simulink model "drone_main_dynamixal"  (R2023b)
settings: Solver=FixedStepAuto  StartTime=0.0  StopTime=inf  FixedStep=0.001  RelTol=1e-3
model workspace: external: MATLAB File drone_DataFile.m (data not in the file)
values from neighbouring files (symbols this model uses):
  coefthrust = 5.7199 / (max_prop^2)    (= 5.7199e-06)    [parameters.m]    (also in parameters.mat)
  coeftorque = 0.4008 / (max_prop^2)    (= 4.008e-07)    [parameters.m]    (also in parameters.mat)
  controlmatrix = pinv(controlmatrix)    [parameters.m]    (also in parameters.mat = [121408.493932 121408.493932 -121408.493932 -121408.493932 -)
  g = 9.8067    [parameters.m]    (also in parameters.mat)
  I = [0.0283    0.0003    0.0072 ... (first row only)    [parameters.m]    (also in parameters.mat = [0.0283  0.0003  0.0072; 0.0003  0.521  -0.0001; 0.0072  -0.)
  M =     [parameters.mat]
  m = pinv(mixmatrix)*b    [test.m]
  max_prop = 1000    [parameters.m]    (also in parameters.mat)
  poly_traj = pTraj    [trajectory.m]
  route = [0 0 1 0.5*pi ... (first row only)    [parameters.m]    (also in parameters.mat = [0 0 -3 -3 -3 3 0 3 3 4 4 4 ... (24 elements, 6x4)])
  smiData = struct    [drone_DataFile.m]
  total_mass = 2.1309    [parameters.m]    (also in parameters.mat)
undefined symbols (not defined in the file or in its folder): mass_total, X, Y, Z
libraries: sm_lib x173, slpidlib x90, nesl_utility x72, fl_lib x32, slctrl_autotuning x21, quadcopter_library x8, sdl_lib x8, simulink x3
(part 1 of 19)
settings Model: Creator=karl  LastModifiedBy=karl
settings SolverCC: ZeroCrossAlgorithm=Adaptive
settings DebuggingCC: MaskedZcDiagnostic=none  IgnoredZcDiagnostic=none
settings ExplorerConfigSet: InternalSimMechanicsExplorerSettings="<ExplorerConfiguration><canonicalview>default</canonicalview><AnimationSetting><BasePlaybackSpeed>1.0</BasePlaybackSpeed><PlaybackSpeedFactor>1.0</PlaybackSpeedFactor></AnimationSetting><TilePanel><TileInfo><Tiles Columns=\"1\" Count=\"1\" Rows=\"1\"><Column Weight=\"1\"/><Row Weight=\"1\"/><Tile Height=\"1\" Width=\"1\" X=\"0\" Y=\"0\"/></Tiles></TileInfo><SceneInfo><SceneViewer><BGColor><R>0.60000002384185791</R><G>0.60000002384185791</G><B>0.60000002384185791</B></BGColor><Camera><DoPerspective>on</DoPerspective><Position><X>2.81198467739789759</X><Y>2.16442511828485351</Y><Z>2.00493354781460198</Z></Position><Center><X>3.04927914831391655</X><Y>4.00827432510628157</Y><Z>0.998712364972069055</Z></Center><Up><X>0</X><Y>-2.22044604925031308e-16</Y><Z>1</Z></Up><ViewLimDist>1</ViewLimDist><YLim>0.466307658154998583</YLim><XLim>0.670479471373142677</XLim></Camera></SceneViewer></SceneInfo></TilePanel><MechEditorPanel><Cameras><Camera><Id>Camera1</Id><Value><Name>Camera1</Name><NativeCamera><PositionTrackingFeature>plant.camera_Frame.R</PositionTrackingFeature><CenterTrackingFeature>plant.centerbody.F6</CenterTrackingFeature><UpVectorTrackingFeature>plant.Cartesian_Joint.F</UpVectorTrackingFeature><CenterTrackingOrigin>on</CenterTrackingOrigin><UpVectorTrackingDirection>-Y</UpVectorTrackingDirection></NativeCamera></Value></Camera></Cameras><GfxPanelCameraMap><MapElement CameraMLId=\"Camera1\" GfxPanelIndex=\"0\"/></GfxPanelCameraMap><VideoCreator><PlaybackSpeedRatio>1.0</PlaybackSpeedRatio><FrameRate>60</FrameRate><VideoFormat>MPEG-4</VideoFormat><FrameSize>[1920 1080]</FrameSize></VideoCreator></MechEditorPanel></ExplorerConfiguration>"

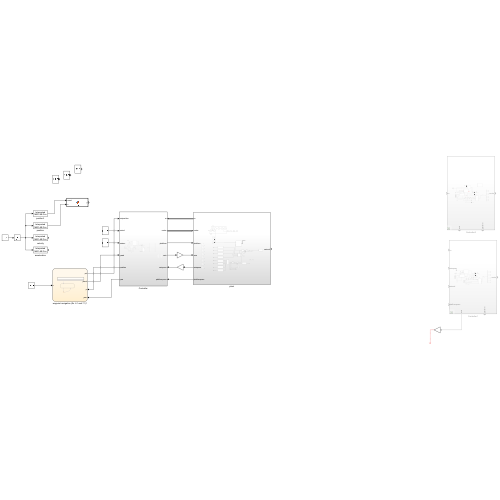
[thumbnail: Simulink's stored preview of the top-level diagram]
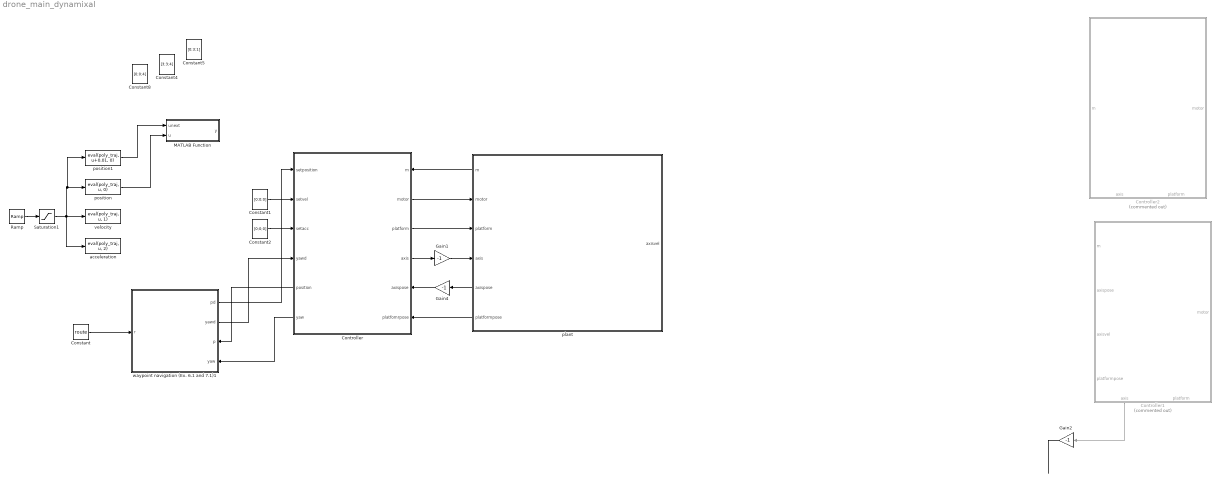
== system drone_main_dynamixal ==
  Constant : Constant  Value=route
  Constant1 : Constant  Value=[0;0;0]
  Constant2 : Constant  Value=[0;0;0]
  Constant4 : Constant  Value=[3;3;4]
  Constant5 : Constant  Value=[0;3;1]
  Constant8 : Constant  Value=[0;0;4]
  Controller : Subsystem
      settings: PortSchema="{\"entries\":[{\"content\":{\"sides\":[{\"content\":{\"connectorIds\":[\"In1\",\"In2\",\"In3\",\"In4\",\"Out4\",\"Out5\"]},\"type\":\"ConnectorPlacement.EquallySpacedRectSide\",\"uuid\":\"efd116df-0710-4bc4-bd30-46d2282b54a0\"},{\"content\":{\"connectorIds\":[\"In5\",\"Out1\",\"Out2\",\"Out3\",\"In6\",\"In7\"],\"side\":\"RIGHT\"},\"type\":\"ConnectorPlacement.EquallySpacedRectSide\",\"uuid\":\"42a0262b-89db-4dee-9ad3-14016f8ac5f1\"},{\"content\":{\"side\":\"TOP\"},\"type\":\"ConnectorPlacement.EquallySpacedRectSide\",\"uuid\":\"e37570b1-13d5-473e-a4a2-7c37e0d0ffe3\"},{\"content\":{\"side\":\"BOTTOM\"},\"type\":\"ConnectorPlacement.EquallySpacedRectSide\",\"uuid\":\"fd86b602-742f-417b-a2c4-bd46caad86d3\"}]},\"type\":\"ConnectorPlacement.EquallySpacedConnector\",\"uuid\":\"c2e19d15-eb80-41e4-99c2-17f1e388988e\"}],\"packageUris\":[\"http://schema.mathworks.com/mf0/Connector/R2020b\"],\"version\":\"1.0\"}"
  Controller1 : Subsystem  Commented=on
      settings: PortSchema="{\"entries\":[{\"content\":{\"sides\":[{\"content\":{\"connectorIds\":[\"In1\",\"In2\",\"In3\",\"In4\"]},\"type\":\"ConnectorPlacement.EquallySpacedRectSide\",\"uuid\":\"efd116df-0710-4bc4-bd30-46d2282b54a0\"},{\"content\":{\"connectorIds\":[\"Out1\"],\"side\":\"RIGHT\"},\"type\":\"ConnectorPlacement.EquallySpacedRectSide\",\"uuid\":\"42a0262b-89db-4dee-9ad3-14016f8ac5f1\"},{\"content\":{\"side\":\"TOP\"},\"type\":\"ConnectorPlacement.EquallySpacedRectSide\",\"uuid\":\"e37570b1-13d5-473e-a4a2-7c37e0d0ffe3\"},{\"content\":{\"connectorIds\":[\"Out2\",\"Out3\"],\"side\":\"BOTTOM\"},\"type\":\"ConnectorPlacement.EquallySpacedRectSide\",\"uuid\":\"fd86b602-742f-417b-a2c4-bd46caad86d3\"}]},\"type\":\"ConnectorPlacement.EquallySpacedConnector\",\"uuid\":\"c2e19d15-eb80-41e4-99c2-17f1e388988e\"}],\"packageUris\":[\"http://schema.mathworks.com/mf0/Connector/R2020b\"],\"version\":\"1.0\"}"
  Controller2 : Subsystem  Commented=on
      settings: PortSchema="{\"entries\":[{\"content\":{\"sides\":[{\"content\":{\"connectorIds\":[\"In1\"]},\"type\":\"ConnectorPlacement.EquallySpacedRectSide\",\"uuid\":\"efd116df-0710-4bc4-bd30-46d2282b54a0\"},{\"content\":{\"connectorIds\":[\"Out1\"],\"side\":\"RIGHT\"},\"type\":\"ConnectorPlacement.EquallySpacedRectSide\",\"uuid\":\"42a0262b-89db-4dee-9ad3-14016f8ac5f1\"},{\"content\":{\"side\":\"TOP\"},\"type\":\"ConnectorPlacement.EquallySpacedRectSide\",\"uuid\":\"e37570b1-13d5-473e-a4a2-7c37e0d0ffe3\"},{\"content\":{\"connectorIds\":[\"Out2\",\"Out3\"],\"side\":\"BOTTOM\"},\"type\":\"ConnectorPlacement.EquallySpacedRectSide\",\"uuid\":\"fd86b602-742f-417b-a2c4-bd46caad86d3\"}]},\"type\":\"ConnectorPlacement.EquallySpacedConnector\",\"uuid\":\"c2e19d15-eb80-41e4-99c2-17f1e388988e\"}],\"packageUris\":[\"http://schema.mathworks.com/mf0/Connector/R2020b\"],\"version\":\"1.0\"}"
  Gain1 : Gain  Gain=-1
  Gain2 : Gain  Gain=-1
  Gain4 : Gain  Gain=-1
  MATLAB Function : MATLAB Function  TreatAsAtomicUnit=on
  Ramp : simulink/Sources/Ramp  slope=1  start=0  InitialOutput=0
  Saturation1 : Saturate  UpperLimit=knots(end)  LowerLimit=0
  acceleration : MATLABFcn  MATLABFcn=eval(poly_traj, u, 2)  OutputDimensions=[3 1]  Output1D=off
  plant : Subsystem
      settings: PortSchema="{\"entries\":[{\"content\":{\"sides\":[{\"content\":{\"connectorIds\":[\"Out2\",\"In1\",\"In2\",\"In3\",\"Out3\",\"Out4\"]},\"type\":\"ConnectorPlacement.EquallySpacedRectSide\",\"uuid\":\"1c064c66-4770-46ed-8bde-fcd9daa0cfea\"},{\"content\":{\"connectorIds\":[\"Out1\"],\"side\":\"RIGHT\"},\"type\":\"ConnectorPlacement.EquallySpacedRectSide\",\"uuid\":\"2bc9ec3c-f7fe-448b-b9a0-aabfb7a731b3\"},{\"content\":{\"side\":\"TOP\"},\"type\":\"ConnectorPlacement.EquallySpacedRectSide\",\"uuid\":\"776f5a84-0136-4a0a-add1-2781f8ebe025\"},{\"content\":{\"side\":\"BOTTOM\"},\"type\":\"ConnectorPlacement.EquallySpacedRectSide\",\"uuid\":\"8fe710a9-ef9a-4b6e-99e6-9612389d5d8d\"}]},\"type\":\"ConnectorPlacement.EquallySpacedConnector\",\"uuid\":\"c1b0af6b-0af1-4f81-9887-9b2d00ee34a0\"}],\"packageUris\":[\"http://schema.mathworks.com/mf0/Connector/R2020b\"],\"version\":\"1.0\"}"
  position : MATLABFcn  MATLABFcn=eval(poly_traj, u, 0)  OutputDimensions=[3 1]  Output1D=off
  position1 : MATLABFcn  MATLABFcn=eval(poly_traj, u+0.01, 0)  OutputDimensions=[3 1]  Output1D=off
  velocity : MATLABFcn  MATLABFcn=eval(poly_traj, u, 1)  OutputDimensions=[3 1]  Output1D=off
  waypoint navigation (Ex. 6.1 and 7.1)1 : Stateflow chart  TreatAsAtomicUnit=on
      settings: PortSchema="{\"entries\":[{\"content\":{\"sides\":[{\"content\":{\"connectorIds\":[\"In1\"]},\"type\":\"ConnectorPlacement.EquallySpacedRectSide\",\"uuid\":\"7c2fff0d-1179-4786-9432-1971d7acd904\"},{\"content\":{\"connectorIds\":[\"Out2\",\"Out1\",\"In3\",\"In2\"],\"side\":\"RIGHT\"},\"type\":\"ConnectorPlacement.EquallySpacedRectSide\",\"uuid\":\"377a8206-b310-41c0-9a17-faf5318c89cb\"},{\"content\":{\"side\":\"TOP\"},\"type\":\"ConnectorPlacement.EquallySpacedRectSide\",\"uuid\":\"b953090a-ffdb-4e30-a5fe-7bef9655f1cf\"},{\"content\":{\"side\":\"BOTTOM\"},\"type\":\"ConnectorPlacement.EquallySpacedRectSide\",\"uuid\":\"03dc7a24-529e-4020-b953-d1c4751c5c80\"}]},\"type\":\"ConnectorPlacement.EquallySpacedConnector\",\"uuid\":\"03bac9f4-6480-492d-9af3-57aec4db8fd8\"}],\"packageUris\":[\"http://schema.mathworks.com/mf0/Connector/R2020b\"],\"version\":\"1.0\"}"
  wires:
  plant/2(m) -> Controller/5(m)
  Controller/2(platform) -> plant/2(platform)
  Controller/3(axis) -> Gain1/1
  Gain1/1 -> plant/3(axis)
  Controller/1(motor) -> plant/1(motor)
  Controller1/2(axis) -> Gain2/1
  Gain2/1 -> ?
  plant/3(axispose) -> Gain4/1
  Gain4/1 -> Controller/6(axispose)
  plant/4(platformpose) -> Controller/7(platfomrpose)
  Constant/1 -> waypoint navigation (Ex. 6.1 and 7.1)1/1(r)
  position/1 -> MATLAB Function/2(u)
  Controller/4(position) -> waypoint navigation (Ex. 6.1 and 7.1)1/3(p)
  waypoint navigation (Ex. 6.1 and 7.1)1/1(yawd) -> Controller/4(yawd)
  Controller/5(yaw) -> waypoint navigation (Ex. 6.1 and 7.1)1/2(yaw)
  Saturation1/1 -> acceleration/1, position1/1, position/1, velocity/1
  Ramp/1 -> Saturation1/1
  position1/1 -> MATLAB Function/1(unext)
  Constant1/1 -> Controller/2(setvel)
  Constant2/1 -> Controller/3(setacc)
  waypoint navigation (Ex. 6.1 and 7.1)1/2(pd) -> Controller/1(setposition)

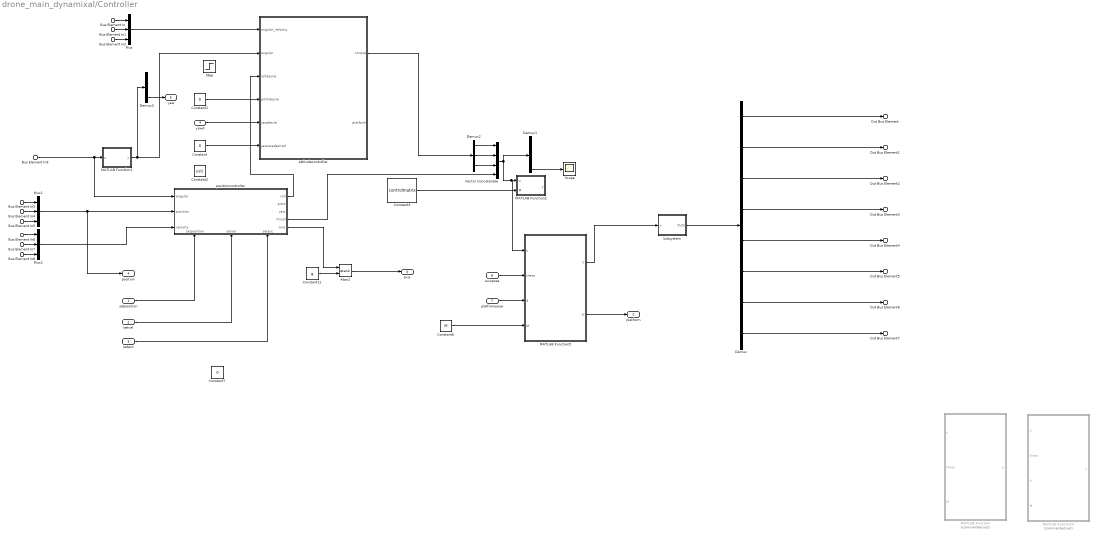
== system drone_main_dynamixal/Controller ==
  setposition : Inport
  setvel : Inport  Port=2
  setacc : Inport  Port=3
  yawd : Inport  Port=4
  Bus Element In : Inport  Port=5  PortName=m  Element=nRoll
  Bus Element In1 : Inport  Port=5  PortName=m  Element=nPitch
  Bus Element In2 : Inport  Port=5  PortName=m  Element=nYaw
  Bus Element In3 : Inport  Port=5  PortName=m  Element=px
  Bus Element In4 : Inport  Port=5  PortName=m  Element=py
  Bus Element In5 : Inport  Port=5  PortName=m  Element=pz
  Bus Element In6 : Inport  Port=5  PortName=m  Element=vx
  Bus Element In7 : Inport  Port=5  PortName=m  Element=vy
  Bus Element In8 : Inport  Port=5  PortName=m  Element=vz
  Bus Element In9 : Inport  Port=5  PortName=m  Element=R
  axispose : Inport  Port=6
  platfomrpose : Inport  Port=7
  Atan2 : Trigonometry  Operator=atan2
  Constant : Constant  Value=0
  Constant1 : Constant  Value=0
  Constant11 : Constant  Value=g
  Constant2 : Constant  Value=pi/2
  Constant3 : Constant  Value=controlmatrix
  Constant6 : Constant  Value=M  OutDataTypeStr=Bus: M_bus
  Constant7 : Constant  Value=0
  Demux : Demux  Outputs=8
  Demux1 : Demux
  Demux2 : Demux  Outputs=3
  Demux3 : Demux  Outputs=3
  MATLAB Function : MATLAB Function  Commented=on  TreatAsAtomicUnit=on
  MATLAB Function1 : MATLAB Function  TreatAsAtomicUnit=on
  MATLAB Function2 : MATLAB Function  TreatAsAtomicUnit=on
  MATLAB Function4 : MATLAB Function  Commented=on  TreatAsAtomicUnit=on
  MATLAB Function5 : MATLAB Function  TreatAsAtomicUnit=on
  Mux : Mux  Inputs=3
  Mux1 : Mux  Inputs=3
  Mux2 : Mux  Inputs=3
  Scope : Scope
  Step : Step  SampleTime=0
  Subsystem : Subsystem
  Vector Concatenate : Concatenate  NumInputs=4
  attitudecontroller : Subsystem
  positioncontroller : Subsystem
      settings: PortSchema="{\"entries\":[{\"content\":{\"sides\":[{\"content\":{\"connectorIds\":[\"In1\",\"In2\",\"In3\"]},\"type\":\"ConnectorPlacement.EquallySpacedRectSide\",\"uuid\":\"8fc0619c-da24-474a-ba81-4a0e6403e529\"},{\"content\":{\"connectorIds\":[\"Out1\",\"Out2\",\"Out3\",\"Out4\",\"Out5\"],\"side\":\"RIGHT\"},\"type\":\"ConnectorPlacement.EquallySpacedRectSide\",\"uuid\":\"3b7bf8fd-1c12-492b-bf3d-80eeb1c43df6\"},{\"content\":{\"side\":\"TOP\"},\"type\":\"ConnectorPlacement.EquallySpacedRectSide\",\"uuid\":\"d4c65c09-2611-4b76-817c-4c3799ca9b05\"},{\"content\":{\"connectorIds\":[\"In4\",\"In5\",\"In6\"],\"side\":\"BOTTOM\"},\"type\":\"ConnectorPlacement.EquallySpacedRectSide\",\"uuid\":\"94af8736-882f-4d33-beaa-402d25cea3b1\"}]},\"type\":\"ConnectorPlacement.EquallySpacedConnector\",\"uuid\":\"0c77d207-25a9-4738-a568-946a6093f630\"}],\"packageUris\":[\"http://schema.mathworks.com/mf0/Connector/R2020b\"],\"version\":\"1.0\"}"
  Out Bus Element : Outport  PortName=motor  Element=Output
  Out Bus Element1 : Outport  PortName=motor  Element=Output1
  Out Bus Element2 : Outport  PortName=motor  Element=Output2
  Out Bus Element3 : Outport  PortName=motor  Element=Output3
  Out Bus Element4 : Outport  PortName=motor  Element=Output4
  Out Bus Element5 : Outport  PortName=motor  Element=Output5
  Out Bus Element6 : Outport  PortName=motor  Element=Output6
  Out Bus Element7 : Outport  PortName=motor  Element=Output7
  platform : Outport  Port=2
  axis : Outport  Port=3
  position : Outport  Port=4
  yaw : Outport  Port=5
  wires:
  Constant3/1 -> MATLAB Function2/2(M)
  Vector Concatenate/1 -> MATLAB Function5/1(u), MATLAB Function2/1(u), Demux1/1
  Bus Element In9/1 -> positioncontroller/1(angular), MATLAB Function1/1(u)
  Subsystem/1(Out1) -> Demux/1
  Mux1/1 -> position/1, positioncontroller/2(position)
  setposition/1 -> positioncontroller/4(setposition)
  Mux/1 -> attitudecontroller/1(angular_velocity)
  attitudecontroller/1(torque) -> Demux2/1
  yawd/1 -> attitudecontroller/5(yawdesire)
  Demux1/4 -> Scope/1
  positioncontroller/4(thrust) -> Vector Concatenate/4
  positioncontroller/1(roll) -> attitudecontroller/3(rolldesire)
  Constant1/1 -> attitudecontroller/4(pitchdesire)
  Mux2/1 -> positioncontroller/3(velocity)
  Bus Element In/1 -> Mux/1
  Bus Element In1/1 -> Mux/2
  Bus Element In2/1 -> Mux/3
  Bus Element In4/1 -> Mux1/2
  Bus Element In5/1 -> Mux1/3
  Bus Element In3/1 -> Mux1/1
  Bus Element In6/1 -> Mux2/1
  Bus Element In8/1 -> Mux2/3
  Bus Element In7/1 -> Mux2/2
  MATLAB Function1/1(y) -> Demux3/1, attitudecontroller/2(angular)
  Demux2/2 -> Vector Concatenate/2
  Demux2/1 -> Vector Concatenate/1
  Demux2/3 -> Vector Concatenate/3
  MATLAB Function5/1(y) -> Subsystem/1(y)
  Constant11/1 -> Atan2/2
  Constant6/1 -> MATLAB Function5/4(M)
  positioncontroller/5(axis) -> Atan2/1
  Constant/1 -> attitudecontroller/6(yawratedesired)
  MATLAB Function5/2(p) -> platform/1
  platfomrpose/1 -> MATLAB Function5/3(d)
  axispose/1 -> MATLAB Function5/2(theta)
  Demux3/3 -> yaw/1
  setacc/1 -> positioncontroller/6(setacc)
  setvel/1 -> positioncontroller/5(setvel)
  Atan2/1 -> axis/1
  Demux/1 -> Out Bus Element/1
  Demux/2 -> Out Bus Element1/1
  Demux/4 -> Out Bus Element3/1
  Demux/3 -> Out Bus Element2/1
  Demux/5 -> Out Bus Element4/1
  Demux/6 -> Out Bus Element5/1
  Demux/7 -> Out Bus Element6/1
  Demux/8 -> Out Bus Element7/1

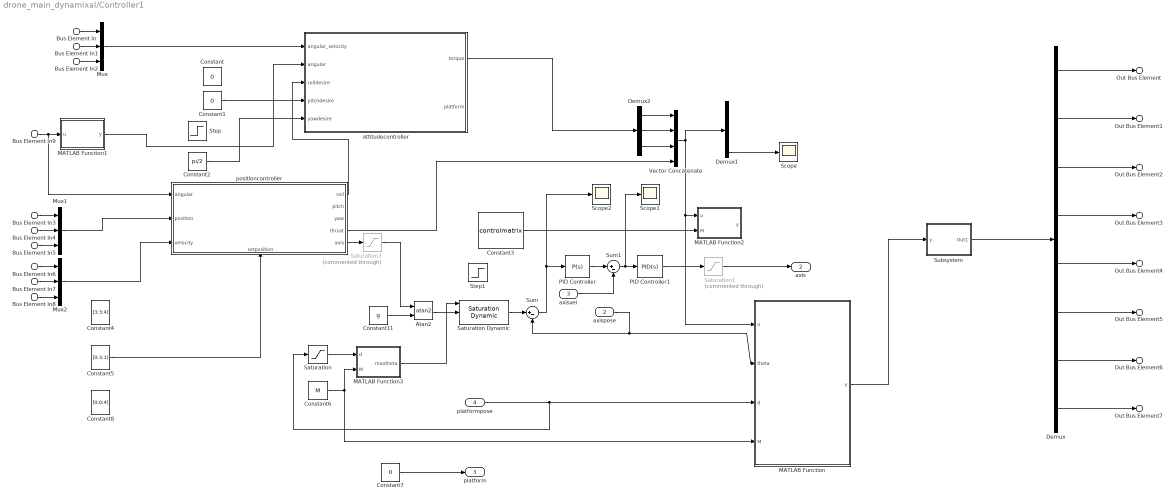
== system drone_main_dynamixal/Controller1 ==
  Bus Element In : Inport  PortName=m  Element=nRoll
  Bus Element In1 : Inport  PortName=m  Element=nPitch
  Bus Element In2 : Inport  PortName=m  Element=nYaw
  Bus Element In3 : Inport  PortName=m  Element=px
  Bus Element In4 : Inport  PortName=m  Element=py
  Bus Element In5 : Inport  PortName=m  Element=pz
  Bus Element In6 : Inport  PortName=m  Element=vx
  Bus Element In7 : Inport  PortName=m  Element=vy
  Bus Element In8 : Inport  PortName=m  Element=vz
  Bus Element In9 : Inport  PortName=m  Element=R
  axispose : Inport  Port=2
  axisvel : Inport  Port=3
  platformpose : Inport  Port=4
  Atan2 : Trigonometry  Operator=atan2
  Constant : Constant  Value=0
  Constant1 : Constant  Value=0
  Constant11 : Constant  Value=g
  Constant2 : Constant  Value=pi/2
  Constant3 : Constant  Value=controlmatrix
  Constant4 : Constant  Value=[3;3;4]
  Constant5 : Constant  Value=[0;3;1]
  Constant6 : Constant  Value=M  OutDataTypeStr=Bus: M_bus
  Constant7 : Constant  Value=0
  Constant8 : Constant  Value=[0;0;4]
  Demux : Demux  Outputs=8
  Demux1 : Demux
  Demux2 : Demux  Outputs=3
  MATLAB Function : MATLAB Function  TreatAsAtomicUnit=on
  MATLAB Function1 : MATLAB Function  TreatAsAtomicUnit=on
  MATLAB Function2 : MATLAB Function  TreatAsAtomicUnit=on
  MATLAB Function3 : MATLAB Function  TreatAsAtomicUnit=on
  Mux : Mux  Inputs=3
  Mux1 : Mux  Inputs=3
  Mux2 : Mux  Inputs=3
  PID Controller : slpidlib/PID Controller  Controller=P  Form=Parallel  TimeDomain=Continuous-time  UseExternalTs=off  SampleTime=-1  IntegratorMethod=Forward Euler  FilterMethod=Forward Euler  ControllerParametersSource=internal  P=1  I=1  UseKiTs=off  D=0  N=100  UseFilter=on  TunerSelectOption=Transfer Function Based (PID Tuner App)  InitialConditionSource=internal  InitialConditionForIntegrator=0  InitialConditionForFilter=0  DifferentiatorICPrevScaledInput=0  ExternalReset=none  TrackingMode=off  Kt=1  LimitOutput=off  SatLimitsSource=internal  UpperSaturationLimit=inf  LowerSaturationLimit=-inf  LinearizeAsGain=on  AntiWindupMode=none  Kb=1  LimitIntegrator=off  UpperIntegratorSaturationLimit=inf  LowerIntegratorSaturationLimit=-inf  POutMin=[]  POutMax=[]  IOutMin=[]  IOutMax=[]  DOutMin=[]  DOutMax=[]  NOutMin=[]  NOutMax=[]  SumOutMin=[]  SumOutMax=[]  SaturationOutMin=[]  SaturationOutMax=[]  PParamMin=[]  PParamMax=[]  IParamMin=[]  IParamMax=[]  DParamMin=[]  DParamMax=[]  NParamMin=[]  NParamMax=[]  KbParamMin=[]  KbParamMax=[]  KtParamMin=[]  KtParamMax=[]  KbOutMin=[]  KbOutMax=[]  KtOutMin=[]  KtOutMax=[]  IntegratorOutMin=[]  IntegratorOutMax=[]  FilterOutMin=[]  FilterOutMax=[]  SumI1OutMin=[]  SumI1OutMax=[]  SumI2OutMin=[]  SumI2OutMax=[]  SumI3OutMin=[]  SumI3OutMax=[]  SumI4OutMin=[]  SumI4OutMax=[]  SumDOutMin=[]  SumDOutMax=[]  DifferentiatorOutMin=[]  DifferentiatorOutMax=[]  FilterDiffOutCoefMin=[]  FilterDiffOutCoefMax=[]  ReciprocalOutMin=[]  ReciprocalOutMax=[]  SumDenOutMin=[]  SumDenOutMax=[]  SumNumOutMin=[]  SumNumOutMax=[]  DivideOutMin=[]  DivideOutMax=[]  UdiffTsProdOutMin=[]  UdiffTsProdOutMax=[]  NTsProdOutMin=[]  NTsProdOutMax=[]  UintegralTsProdOutMin=[]  UintegralTsProdOutMax=[]  UngainTsProdOutMin=[]  UngainTsProdOutMax=[]  ClampingZeroOutDataTypeStr=Inherit: Inherit via back propagation  ClampingZeroOutMin=[]  ClampingZeroOutMax=[]  FilterDenConstantOutDataTypeStr=Inherit: Inherit via back propagation  FilterDenConstantOutMin=[]  FilterDenConstantOutMax=[]  PCopyOutDataTypeStr=Inherit: Inherit via back propagation  PCopyOutMin=[]  PCopyOutMax=[]  NCopyOutDataTypeStr=Inherit: Inherit via back propagation  NCopyOutMin=[]  NCopyOutMax=[]  IntegratorContinuousStateAttributes=''  IntegratorStateMustResolveToSignalObject=off  IntegratorRTWStateStorageClass=Auto  FilterContinuousStateAttributes=''  FilterStateMustResolveToSignalObject=off  FilterRTWStateStorageClass=Auto  ParallelPVariant=InternalParameters  IdealPVariant=Disabled  IVariant=Disabled  DVariant=Disabled  IntegratorVariant=Disabled  SatVariant=Disabled  AWVariant=Disabled  PCopyVariant=Disabled  TRVariant=Disabled  FdbkBlocksVariant=Forward  IdealPFdbkVariant=Disabled  SatFdbkVariant=Disabled  DerivativeFilterVariant=Disabled  NVariant=Disabled  NCopyVariant=Disabled_SignalSpec  FilterICVariant=Disabled  IntegratorICVariant=Disabled  ExternalResetVariant=Disabled  TRSumVariant=Passthrough  SumFdbkVariant=Disabled  SumVariant=Passthrough_P  TsampFilterVariant=InternalTs  TsampNgainVariant=Passthrough  TsampIntegralVariant=Disabled_SignalSpec  ExternalSaturationOutDataTypeStr=Inherit: Same as second input
  PID Controller1 : slpidlib/PID Controller  Controller=PID  Form=Parallel  TimeDomain=Continuous-time  UseExternalTs=off  SampleTime=-1  IntegratorMethod=Forward Euler  FilterMethod=Forward Euler  ControllerParametersSource=internal  P=10  I=10  UseKiTs=off  D=0  N=100  UseFilter=on  TunerSelectOption=Transfer Function Based (PID Tuner App)  InitialConditionSource=internal  InitialConditionForIntegrator=0  InitialConditionForFilter=0  DifferentiatorICPrevScaledInput=0  ExternalReset=none  TrackingMode=off  Kt=1  LimitOutput=off  SatLimitsSource=internal  UpperSaturationLimit=inf  LowerSaturationLimit=-inf  LinearizeAsGain=on  AntiWindupMode=none  Kb=1  LimitIntegrator=off  UpperIntegratorSaturationLimit=inf  LowerIntegratorSaturationLimit=-inf  POutMin=[]  POutMax=[]  IOutMin=[]  IOutMax=[]  DOutMin=[]  DOutMax=[]  NOutMin=[]  NOutMax=[]  SumOutMin=[]  SumOutMax=[]  SaturationOutMin=[]  SaturationOutMax=[]  PParamMin=[]  PParamMax=[]  IParamMin=[]  IParamMax=[]  DParamMin=[]  DParamMax=[]  NParamMin=[]  NParamMax=[]  KbParamMin=[]  KbParamMax=[]  KtParamMin=[]  KtParamMax=[]  KbOutMin=[]  KbOutMax=[]  KtOutMin=[]  KtOutMax=[]  IntegratorOutMin=[]  IntegratorOutMax=[]  FilterOutMin=[]  FilterOutMax=[]  SumI1OutMin=[]  SumI1OutMax=[]  SumI2OutMin=[]  SumI2OutMax=[]  SumI3OutMin=[]  SumI3OutMax=[]  SumI4OutMin=[]  SumI4OutMax=[]  SumDOutMin=[]  SumDOutMax=[]  DifferentiatorOutMin=[]  DifferentiatorOutMax=[]  FilterDiffOutCoefMin=[]  FilterDiffOutCoefMax=[]  ReciprocalOutMin=[]  ReciprocalOutMax=[]  SumDenOutMin=[]  SumDenOutMax=[]  SumNumOutMin=[]  SumNumOutMax=[]  DivideOutMin=[]  DivideOutMax=[]  UdiffTsProdOutMin=[]  UdiffTsProdOutMax=[]  NTsProdOutMin=[]  NTsProdOutMax=[]  UintegralTsProdOutMin=[]  UintegralTsProdOutMax=[]  UngainTsProdOutMin=[]  UngainTsProdOutMax=[]  ClampingZeroOutDataTypeStr=Inherit: Inherit via back propagation  ClampingZeroOutMin=[]  ClampingZeroOutMax=[]  FilterDenConstantOutDataTypeStr=Inherit: Inherit via back propagation  FilterDenConstantOutMin=[]  FilterDenConstantOutMax=[]  PCopyOutDataTypeStr=Inherit: Inherit via back propagation  PCopyOutMin=[]  PCopyOutMax=[]  NCopyOutDataTypeStr=Inherit: Inherit via back propagation  NCopyOutMin=[]  NCopyOutMax=[]  IntegratorContinuousStateAttributes=''  IntegratorStateMustResolveToSignalObject=off  IntegratorRTWStateStorageClass=Auto  FilterContinuousStateAttributes=''  FilterStateMustResolveToSignalObject=off  FilterRTWStateStorageClass=Auto  ParallelPVariant=InternalParameters  IdealPVariant=Disabled  IVariant=InternalParameters  DVariant=InternalParameters  IntegratorVariant=Continuous  SatVariant=Disabled  AWVariant=Passthrough  PCopyVariant=Disabled  TRVariant=Disabled  FdbkBlocksVariant=Forward  IdealPFdbkVariant=Disabled  SatFdbkVariant=Disabled  DerivativeFilterVariant=ContFilter  NVariant=InternalParameters  NCopyVariant=Disabled  FilterICVariant=InternalICsFilter  IntegratorICVariant=InternalICs  ExternalResetVariant=Disabled  TRSumVariant=Passthrough  SumFdbkVariant=Disabled  SumVariant=Sum_PID  TsampFilterVariant=InternalTs  TsampNgainVariant=Passthrough  TsampIntegralVariant=Disabled_SignalSpec  ExternalSaturationOutDataTypeStr=Inherit: Same as second input
  Saturation : Saturate  UpperLimit=0.4  LowerLimit=-0.03
  Saturation Dynamic : simulink/Discontinuities/Saturation Dynamic  OutMin=[]  OutMax=[]  OutDataTypeStr=Inherit: Same as second input  OutDataType=fixdt(1, 16)  OutScaling=2^-10  DoSatur=off
  Saturation1 : Saturate  Commented=through  UpperLimit=1  LowerLimit=-1
  Saturation3 : Saturate  Commented=through  UpperLimit=2*g  LowerLimit=-2*g
  Scope : Scope
  Scope1 : Scope
  Scope2 : Scope
  Step : Step  SampleTime=0
  Step1 : Step  SampleTime=0
  Subsystem : Subsystem
  Sum : Sum  Inputs=|+-
  Sum1 : Sum  Inputs=|+-
  Vector Concatenate : Concatenate  NumInputs=4
  attitudecontroller : Subsystem
  positioncontroller : Subsystem
      settings: PortSchema="{\"entries\":[{\"content\":{\"sides\":[{\"content\":{\"connectorIds\":[\"In1\",\"In2\",\"In3\"]},\"type\":\"ConnectorPlacement.EquallySpacedRectSide\",\"uuid\":\"8fc0619c-da24-474a-ba81-4a0e6403e529\"},{\"content\":{\"connectorIds\":[\"Out1\",\"Out2\",\"Out3\",\"Out4\",\"Out5\"],\"side\":\"RIGHT\"},\"type\":\"ConnectorPlacement.EquallySpacedRectSide\",\"uuid\":\"3b7bf8fd-1c12-492b-bf3d-80eeb1c43df6\"},{\"content\":{\"side\":\"TOP\"},\"type\":\"ConnectorPlacement.EquallySpacedRectSide\",\"uuid\":\"d4c65c09-2611-4b76-817c-4c3799ca9b05\"},{\"content\":{\"connectorIds\":[\"In4\"],\"side\":\"BOTTOM\"},\"type\":\"ConnectorPlacement.EquallySpacedRectSide\",\"uuid\":\"94af8736-882f-4d33-beaa-402d25cea3b1\"}]},\"type\":\"ConnectorPlacement.EquallySpacedConnector\",\"uuid\":\"0c77d207-25a9-4738-a568-946a6093f630\"}],\"packageUris\":[\"http://schema.mathworks.com/mf0/Connector/R2020b\"],\"version\":\"1.0\"}"
  Out Bus Element : Outport  PortName=motor  Element=Output
  Out Bus Element1 : Outport  PortName=motor  Element=Output1
  Out Bus Element2 : Outport  PortName=motor  Element=Output2
  Out Bus Element3 : Outport  PortName=motor  Element=Output3
  Out Bus Element4 : Outport  PortName=motor  Element=Output4
  Out Bus Element5 : Outport  PortName=motor  Element=Output5
  Out Bus Element6 : Outport  PortName=motor  Element=Output6
  Out Bus Element7 : Outport  PortName=motor  Element=Output7
  axis : Outport  Port=2
  platform : Outport  Port=3
  wires:
  Constant3/1 -> MATLAB Function2/2(M)
  Vector Concatenate/1 -> MATLAB Function/1(u), MATLAB Function2/1(u), Demux1/1
  Demux/1 -> Out Bus Element/1
  Bus Element In9/1 -> positioncontroller/1(angular), MATLAB Function1/1(u)
  Demux/2 -> Out Bus Element1/1
  Demux/3 -> Out Bus Element2/1
  Demux/4 -> Out Bus Element3/1
  Demux/5 -> Out Bus Element4/1
  Demux/6 -> Out Bus Element5/1
  Demux/7 -> Out Bus Element6/1
  Demux/8 -> Out Bus Element7/1
  Subsystem/1(Out1) -> Demux/1
  Mux1/1 -> positioncontroller/2(position)
  Constant5/1 -> positioncontroller/4(setposition)
  Mux/1 -> attitudecontroller/1(angular_velocity)
  attitudecontroller/1(torque) -> Demux2/1
  Constant2/1 -> attitudecontroller/5(yawdesire)
  Demux1/4 -> Scope/1
  positioncontroller/4(thrust) -> Vector Concatenate/4
  positioncontroller/1(roll) -> attitudecontroller/3(rolldesire)
  Constant1/1 -> attitudecontroller/4(pitchdesire)
  Mux2/1 -> positioncontroller/3(velocity)
  Bus Element In/1 -> Mux/1
  Bus Element In1/1 -> Mux/2
  Bus Element In2/1 -> Mux/3
  Bus Element In4/1 -> Mux1/2
  Bus Element In5/1 -> Mux1/3
  Bus Element In3/1 -> Mux1/1
  Bus Element In6/1 -> Mux2/1
  Bus Element In8/1 -> Mux2/3
  Bus Element In7/1 -> Mux2/2
  MATLAB Function1/1(y) -> attitudecontroller/2(angular)
  Demux2/2 -> Vector Concatenate/2
  Demux2/1 -> Vector Concatenate/1
  Demux2/3 -> Vector Concatenate/3
  MATLAB Function/1(y) -> Subsystem/1(y)
  positioncontroller/5(axis) -> Saturation3/1
  Constant11/1 -> Atan2/2
  Constant6/1 -> MATLAB Function/4(M), MATLAB Function3/2(M)
  Saturation/1 -> MATLAB Function3/1(d)
  Saturation Dynamic/1 -> Sum/1
  Saturation3/1 -> Atan2/1
  Atan2/1 -> Saturation Dynamic/2
  MATLAB Function3/1(maxtheta) -> Saturation Dynamic/1
  platformpose/1 -> Saturation/1, MATLAB Function/3(d)
  axispose/1 -> MATLAB Function/2(theta), Sum/2
  Sum/1 -> Scope2/1, PID Controller/1
  PID Controller1/1 -> Saturation1/1
  PID Controller/1 -> Sum1/1
  axisvel/1 -> Sum1/2
  Sum1/1 -> Scope1/1, PID Controller1/1
  Saturation1/1 -> axis/1
  Constant7/1 -> platform/1

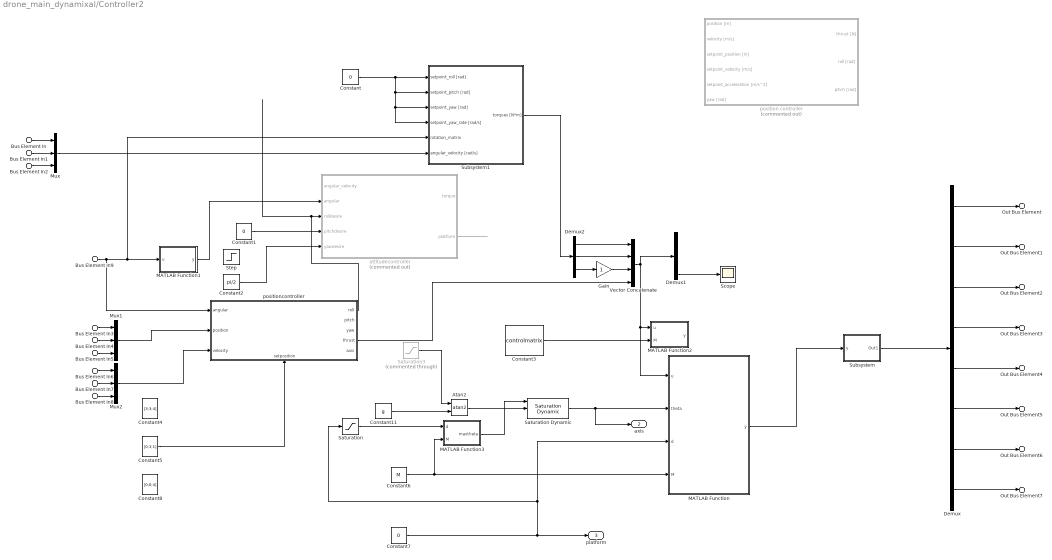
== system drone_main_dynamixal/Controller2 ==
  Bus Element In : Inport  PortName=m  Element=nRoll
  Bus Element In1 : Inport  PortName=m  Element=nPitch
  Bus Element In2 : Inport  PortName=m  Element=nYaw
  Bus Element In3 : Inport  PortName=m  Element=px
  Bus Element In4 : Inport  PortName=m  Element=py
  Bus Element In5 : Inport  PortName=m  Element=pz
  Bus Element In6 : Inport  PortName=m  Element=vx
  Bus Element In7 : Inport  PortName=m  Element=vy
  Bus Element In8 : Inport  PortName=m  Element=vz
  Bus Element In9 : Inport  PortName=m  Element=R
  Atan2 : Trigonometry  Operator=atan2
  Constant : Constant  Value=0
  Constant1 : Constant  Value=0
  Constant11 : Constant  Value=g
  Constant2 : Constant  Value=pi/2
  Constant3 : Constant  Value=controlmatrix
  Constant4 : Constant  Value=[3;3;4]
  Constant5 : Constant  Value=[0;3;1]
  Constant6 : Constant  Value=M  OutDataTypeStr=Bus: M_bus
  Constant7 : Constant  Value=0
  Constant8 : Constant  Value=[0;0;4]
  Demux : Demux  Outputs=8
  Demux1 : Demux
  Demux2 : Demux  Outputs=3
  Gain : Gain
  MATLAB Function : MATLAB Function  TreatAsAtomicUnit=on
  MATLAB Function1 : MATLAB Function  TreatAsAtomicUnit=on
  MATLAB Function2 : MATLAB Function  TreatAsAtomicUnit=on
  MATLAB Function3 : MATLAB Function  TreatAsAtomicUnit=on
  Mux : Mux  Inputs=3
  Mux1 : Mux  Inputs=3
  Mux2 : Mux  Inputs=3
  Saturation : Saturate  UpperLimit=0.4  LowerLimit=-0.03
  Saturation Dynamic : simulink/Discontinuities/Saturation Dynamic  OutMin=[]  OutMax=[]  OutDataTypeStr=Inherit: Same as second input  OutDataType=fixdt(1, 16)  OutScaling=2^-10  DoSatur=off
  Saturation3 : Saturate  Commented=through  UpperLimit=2*g  LowerLimit=-2*g
  Scope : Scope
  Step : Step  SampleTime=0
  Subsystem : Subsystem
  Subsystem1 : Subsystem
      mask Display: image('$imagefile'); % Use "Edit Image" on toolstrip to change.
  Vector Concatenate : Concatenate  NumInputs=4
  attitudecontroller : Subsystem  Commented=on
  position controller : Subsystem  Commented=on
      mask Display: image('$imagefile'); % Use "Edit Image" on toolstrip to change.
  positioncontroller : Subsystem
      settings: PortSchema="{\"entries\":[{\"content\":{\"sides\":[{\"content\":{\"connectorIds\":[\"In1\",\"In2\",\"In3\"]},\"type\":\"ConnectorPlacement.EquallySpacedRectSide\",\"uuid\":\"8fc0619c-da24-474a-ba81-4a0e6403e529\"},{\"content\":{\"connectorIds\":[\"Out1\",\"Out2\",\"Out3\",\"Out4\",\"Out5\"],\"side\":\"RIGHT\"},\"type\":\"ConnectorPlacement.EquallySpacedRectSide\",\"uuid\":\"3b7bf8fd-1c12-492b-bf3d-80eeb1c43df6\"},{\"content\":{\"side\":\"TOP\"},\"type\":\"ConnectorPlacement.EquallySpacedRectSide\",\"uuid\":\"d4c65c09-2611-4b76-817c-4c3799ca9b05\"},{\"content\":{\"connectorIds\":[\"In4\"],\"side\":\"BOTTOM\"},\"type\":\"ConnectorPlacement.EquallySpacedRectSide\",\"uuid\":\"94af8736-882f-4d33-beaa-402d25cea3b1\"}]},\"type\":\"ConnectorPlacement.EquallySpacedConnector\",\"uuid\":\"0c77d207-25a9-4738-a568-946a6093f630\"}],\"packageUris\":[\"http://schema.mathworks.com/mf0/Connector/R2020b\"],\"version\":\"1.0\"}"
  Out Bus Element : Outport  PortName=motor  Element=Output
  Out Bus Element1 : Outport  PortName=motor  Element=Output1
  Out Bus Element2 : Outport  PortName=motor  Element=Output2
  Out Bus Element3 : Outport  PortName=motor  Element=Output3
  Out Bus Element4 : Outport  PortName=motor  Element=Output4
  Out Bus Element5 : Outport  PortName=motor  Element=Output5
  Out Bus Element6 : Outport  PortName=motor  Element=Output6
  Out Bus Element7 : Outport  PortName=motor  Element=Output7
  axis : Outport  Port=2
  platform : Outport  Port=3
  wires:
  Constant3/1 -> MATLAB Function2/2(M)
  Vector Concatenate/1 -> MATLAB Function/1(u), MATLAB Function2/1(u), Demux1/1
  Demux/1 -> Out Bus Element/1
  Bus Element In9/1 -> positioncontroller/1(angular), Subsystem1/5(rotation_matrix), MATLAB Function1/1(u)
  Demux/2 -> Out Bus Element1/1
  Demux/3 -> Out Bus Element2/1
  Demux/4 -> Out Bus Element3/1
  Demux/5 -> Out Bus Element4/1
  Demux/6 -> Out Bus Element5/1
  Demux/7 -> Out Bus Element6/1
  Demux/8 -> Out Bus Element7/1
  Subsystem/1(Out1) -> Demux/1
  Mux1/1 -> positioncontroller/2(position)
  Constant5/1 -> positioncontroller/4(setposition)
  Mux/1 -> Subsystem1/6(angular_velocity [rad/s])
  Subsystem1/1(torques [N*m]) -> Demux2/1
  Constant2/1 -> attitudecontroller/5(yawdesire)
  Demux1/4 -> Scope/1
  positioncontroller/4(thrust) -> Vector Concatenate/4
  positioncontroller/1(roll) -> attitudecontroller/3(rolldesire)
  Constant1/1 -> attitudecontroller/4(pitchdesire)
  Mux2/1 -> positioncontroller/3(velocity)
  Bus Element In/1 -> Mux/1
  Bus Element In1/1 -> Mux/2
  Bus Element In2/1 -> Mux/3
  Bus Element In4/1 -> Mux1/2
  Bus Element In5/1 -> Mux1/3
  Bus Element In3/1 -> Mux1/1
  Bus Element In6/1 -> Mux2/1
  Bus Element In8/1 -> Mux2/3
  Bus Element In7/1 -> Mux2/2
  MATLAB Function1/1(y) -> attitudecontroller/2(angular)
  Demux2/2 -> Vector Concatenate/2
  Demux2/1 -> Vector Concatenate/1
  Demux2/3 -> Gain/1
  MATLAB Function/1(y) -> Subsystem/1(y)
  ? -> Saturation3/1
  Constant11/1 -> Atan2/2
  Constant6/1 -> MATLAB Function3/2(M), MATLAB Function/4(M)
  Saturation/1 -> MATLAB Function3/1(d)
  Saturation Dynamic/1 -> axis/1, MATLAB Function/2(theta)
  Saturation3/1 -> Atan2/1
  Atan2/1 -> Saturation Dynamic/2
  MATLAB Function3/1(maxtheta) -> Saturation Dynamic/1
  attitudecontroller/2(platform) -> ?
  Constant7/1 -> MATLAB Function/3(d), Saturation/1, platform/1
  Constant/1 -> Subsystem1/1(setpoint_roll [rad]), Subsystem1/4(setpoint_yaw_rate [rad/s]), Subsystem1/3(setpoint_yaw [rad]), Subsystem1/2(setpoint_pitch [rad])
  Gain/1 -> Vector Concatenate/3
